simulink model "model_1"  (R2014b)
settings: Solver=ode45  StartTime=0.0  StopTime=50  MaxStep=0.1  RelTol=1e-3
settings Model: Creator=Shane Reynolds  LastModifiedBy=Shane Reynolds

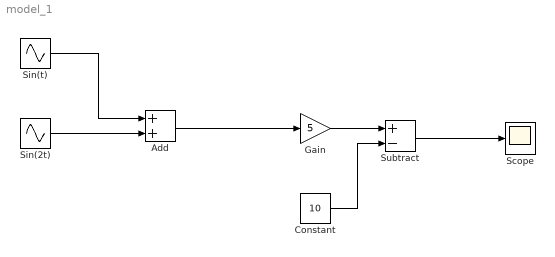
== system model_1 ==
  Add : Sum
  Constant : Constant  Value=10
  Gain : Gain  Gain=5
  Scope : Scope
  Sin(2t) : Sin  Frequency=2  SampleTime=0
  Sin(t) : Sin  SampleTime=0
  Subtract : Sum  Inputs=+-
  wires:
  Sin(2t)/1 -> Add/2
  Sin(t)/1 -> Add/1
  Add/1 -> Gain/1
  Gain/1 -> Subtract/1
  Subtract/1 -> Scope/1
  Constant/1 -> Subtract/2
